simulink model "SVC_Simulation_new"  (R2024a)
settings: Solver=FixedStepDiscrete  StartTime=0.0  StopTime=0.6  FixedStep=Ts  RelTol=1e-3
model workspace (MAT data in the model file):
  Bcap = Simulink.Parameter
  Bcap.Value = 3.23
  Bcap.Complexity = 'real'
  Bcap.Dimensions = [1 1]
  Bcap.DataType = 'auto'
  Bind = Simulink.Parameter
  Bind.Value = -1.04
  Bind.Complexity = 'real'
  Bind.Dimensions = [1 1]
  Bind.DataType = 'auto'
  Bmax = Simulink.Parameter
  Bmax.Value = 3.23
  Bmax.Complexity = 'real'
  Bmax.Dimensions = [1 1]
  Bmax.DataType = 'auto'
  Bmin = Simulink.Parameter
  Bmin.Value = -1.04
  Bmin.Complexity = 'real'
  Bmin.Dimensions = [1 1]
  Bmin.DataType = 'auto'
  Bmmin_max = 0
  Bref = 0
  Ki = Simulink.Parameter
  Ki.Value = 800
  Ki.Complexity = 'real'
  Ki.Dimensions = [1 1]
  Ki.DataType = 'auto'
  Kp = Simulink.Parameter
  Kp.Value = 0
  Kp.Complexity = 'real'
  Kp.Dimensions = [1 1]
  Kp.DataType = 'auto'
  KpKi = 0
  OpMode = 1
  Ts = 5e-05
  Vref = 0
  Xs = 0
undefined symbols (not defined in the file or in its folder): D1, Delta, DiscIntNeverNeededParam
libraries: spsThreePhaseVIMeasurementLib x2, spsThreePhaseSeriesRLCLoadLib x1, spsThreePhaseTransformerTwoWindingsLib x1, spsThreePhaseSeriesRLCBranchLib x1, spsGroundLib x1, spsPLL3phLib x1, spsPositiveSequencePLLDrivenLib x1, spsThreePhaseProgrammableVoltageSourceLib x1, spsStairGeneratorLib x1, sps_lib x1
settings Model: ParameterArgumentNames=Bmmin_max,Bref,KpKi,OpMode,Ts,Vref,Xs  Creator=E370_  LastModifiedBy=E370_

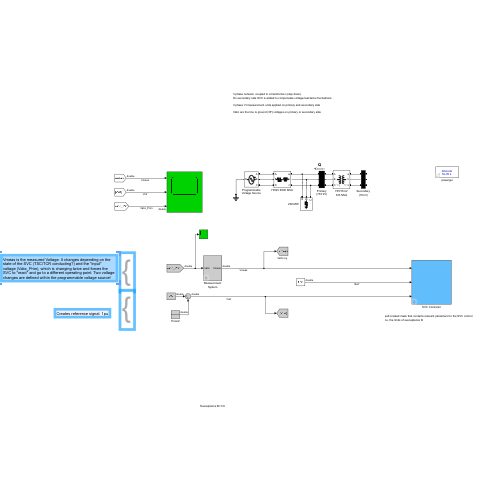
[thumbnail: Simulink's stored preview of the top-level diagram]
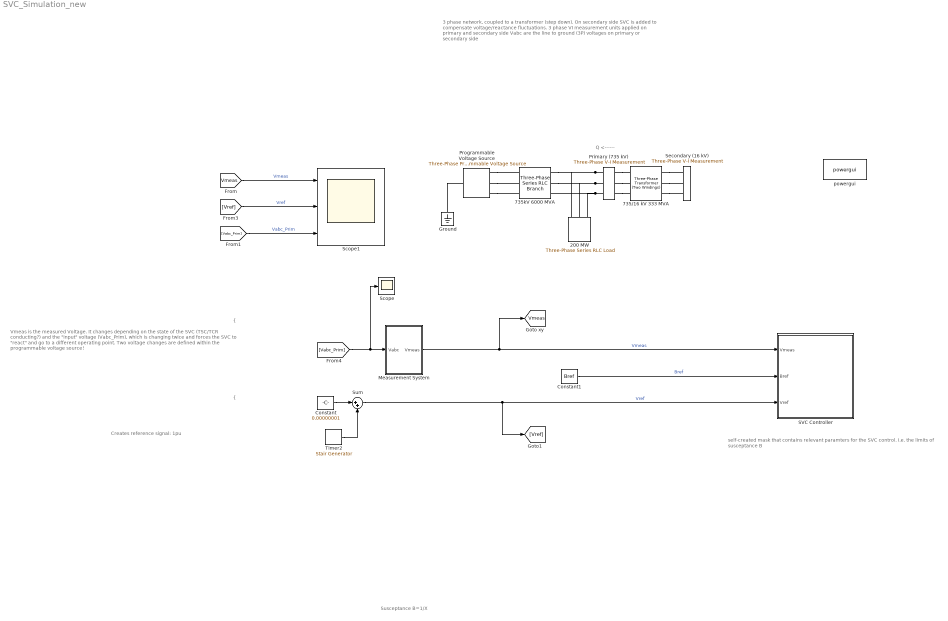
== system SVC_Simulation_new ==
  note: {
  note: Vmeas is the measured Voltage. It changes depending on the state of the SVC (TSC/TCR conducting?) and the "input" voltage (Vabc_Prim), which is changing twice and forces the SVC to "react" and go to a different operating point. Two voltage changes are defined within the programmable voltage source!
  note: self-created mask that contains relevant paramters for the SVC control.
      | I.e. the limits of susceptance B
  note: Susceptance B=1/X
  note: Creates reference signal: 1pu
  note: 3 phase network, coupled to a transformer (step down).
      | On secondary side SVC is added to compensate voltage/reactance fluctuations.
      |
      | 3 phase VI measurement units applied on primary and secondary side
      |
      | Vabc are the line to ground (3P) voltages on primary or secondary side
  note: Q
      | <------
  note: {
  200 MW : spsThreePhaseSeriesRLCLoadLib/Three-Phase Series RLC Load  LConnTagsString=A|B|C  Configuration=Y (grounded)  NominalVoltage=735e3  Vabc=[1e3 1e3 1e3]  Vabcp=[1e3 1e3 1e3]  NominalFrequency=60  UnbalancedPower=off  ActivePower=200e6  InductivePower=0  CapacitivePower=0  Pabc=[10e3 9e3 11e3]  QLabc=[100 90 110]  QCabc=[100 90 110]  Pabcp=[10e3 9e3 11e3]  QLabcp=[100 90 110]  QCabcp=[100 90 110]  Measurements=None  LoadType=constant Z
  735/16 kV 333 MVA : spsThreePhaseTransformerTwoWindingsLib/Three-Phase Transformer (Two Windings)  Winding1Connection=Yg  Winding2Connection=Delta (D1)  CoreType=Three single-phase transformers  SetSaturation=off  Hysteresis=off  DataFile='hysteresis'  SetInitialFlux=off  Measurements=None  UNITS=pu  NominalPower=[333e6 , 60 ]  Winding1=[735e3 , 0.15/30/2 , 0.15*0.7]  Winding2=[ 16e3 , 0.15/30/2, 0.15*0.3]  Rm=500  Lm=500  L0=0.5  Saturation="[ 0,0  ;  0.005,1.2  ;  1.0,1.4 ]"  InitialFluxes=[ 0.8 , -0.8 , 0.7 ]  BreakLoop=off  DiscreteSolver=Trapezoidal iterative  DataType=off  TransfoNumber=0
  "735kV 6000 MVA " : spsThreePhaseSeriesRLCBranchLib/Three-Phase Series RLC Branch  LConnTagsString=A|B|C  RConnTagsString=A|B|C  BranchType=RL  Resistance=735e3^2/6000e6/10  Inductance=735e3^2/6000e6/(2*pi*60)  Capacitance=1.0  Measurements=None
  Constant : Constant  Value=0.00000001
  Constant1 : Constant  Value=Bref
  Ground : spsGroundLib/Ground  LConnTagsString=a
  Measurement System : Subsystem  mask(SVC measurement system){Vnom=735e3, ParI=[735e3*0.9998 0 60], Ts=Ts}
      mask prompts: Vnom "Nominal voltage (volts rms ph-ph)"; ParI "Initial input: [ Mag (volts rms ph-ph)  Phase (degree) Freq (Hz) ]"; Ts "Sample time:"
      mask init:
      | Mag_Init=ParI(1)/Vnom;
      | Phase_Init=ParI(2);
      | Freq_Init=ParI(3);
  Primary (735 kV) : spsThreePhaseVIMeasurementLib/Three-Phase V-I Measurement  VoltageMeasurement=phase-to-ground  SetLabelV=on  LabelV=Vabc_Prim  Vpu=on  VpuLL=off  CurrentMeasurement=yes  SetLabelI=on  LabelI=Iabc_Prim  Ipu=on  Pbase=100e6  Vbase=735e3  OutputType=Magnitude  PhasorSimulation=off  PSBequivalent=0
  Programmable Voltage Source : spsThreePhaseProgrammableVoltageSourceLib/Three-Phase Programmable Voltage Source  PositiveSequence="[1.004*735e3 0  60]"  VariationEntity=Amplitude  VariationType=Table of time-amplitude pairs  VariationTypeAlt=Step  VariationStep=-0.3  VariationRate=0.5  VariationMagnitude=0.4  VariationFrequency=2  VariationTiming=[0.1 1.2]  VariationPhaseA=off  Amplitudes=[1.0 1.025 0.93 1.0 ]  TimeValues=[0 0.1 0.4 0.7]  HarmonicGeneration=off  HarmonicA=[3 0.2 -25 0]  HarmonicB="[2 0.15  35 2]"  Timing="[0.1  0.6]"  BusType=swing  Pref=0  Qref=0  Qmin=-inf  Qmax=inf
  SVC Controller : Subsystem  mask{Vref=1.0, KpKi=[ 0 800 ], Xs=0.01, Bmin_max=[ -1.04 3.23], Bref=0, Ts=Ts}
      mask prompts: Vref "reference voltage (pu):"; KpKi "regulator gains [Kp Ki]:"; Xs "droop"; Bmin_max "Min. and max. primary susceptances [ Bind Bcap] (pu/100MVA):"; Bref "susceptance Bref (pu/100MVA) (Var control mode):"; Ts "sample time (s):"
      mask DialogControl Control2 Prompt: Voltage Regulation Mode
      mask Display: color('red');
  Scope : Scope
  Scope1 : Scope  NumInputPorts=3
  Secondary (16 kV) : spsThreePhaseVIMeasurementLib/Three-Phase V-I Measurement  VoltageMeasurement=phase-to-phase  SetLabelV=on  LabelV=Vabc_Sec  Vpu=on  VpuLL=off  CurrentMeasurement=no  SetLabelI=off  LabelI=Iabc_Sec  Ipu=off  Pbase=100e6  Vbase=16e3  OutputType=Magnitude  PhasorSimulation=off  PSBequivalent=0
  Sum : Sum  Inputs=|++  SaturateOnIntegerOverflow=on
  Timer2 : spsStairGeneratorLib/Stair Generator  t="[ 0  0.4  0.6 ]"  e=[1 1 1 ]  Ts=Ts
  powergui : sps_lib/powergui  Priority=1  SimulationMode=Discrete  SampleTime=Ts  frequency=60  Iterations=50  frequencyindice=60  Pbase=100e6  ErrMax=1e-4  UnitsV=kV  UnitsW=MW  buscounter=0  FunctionMessages=off  echomessages=off  EnableUseOfTLC=off  CurrentSourceSwitches=off  DisableSnubberDevices=off  DisableRonSwitches=off  DisableVfSwitches=off  DisplayEquations=off  AutomaticDiscreteSolvers=off  SolverType=Tustin/Backward Euler (TBE)  Interpol=off  ExternalGateDelay=off  methode=off  Ts=100  x0status=blocks  SPID=on  SwTol=0  HookPort=off  NonlinearTolerance=1e-4  nMaxIteration=100  ContinueOnMaxIteration=off  RestoreLinks=warning  ResistiveCurrentMeasurement=off  Frange=[0:2:500]  Ylog=off  Xlog=on  ShowGrid=off  save=off  variable=ZData  structure=0  ZoomFFT=off  StartTime=0.0  cycles=1  DisplayStyle=1  fundamental=60  FreqAxis=off  MaxFrequency=1000  frequencyindicesteady=1  RmsSteady=1  display=off
  tag scope: Vmeas=global
  wires:
  [Vabc_Prim] -> Scope/1, Measurement System/1(Vabc)
  Timer2/1 -> Sum/2
  Constant/1 -> Sum/1
  [Vref] -> Scope1/2  "Vref"
  Constant1/1 -> SVC Controller/2(Bref)  "Bref"
  Measurement System/1(Vmeas) -> [Vmeas], SVC Controller/1(Vmeas)  "Vmeas"
  [Vmeas] -> Scope1/1  "Vmeas"
  Sum/1 -> SVC Controller/3(Vref), [Vref]  "Vref"
  [Vabc_Prim] -> Scope1/3  "Vabc_Prim"
  connections:
  Primary (735 kV)/LConn2 -- 200 MW/LConn2 -- "735kV 6000 MVA "/RConn2
  Primary (735 kV)/LConn3 -- 200 MW/LConn3 -- "735kV 6000 MVA "/RConn3
  Primary (735 kV)/LConn1 -- 200 MW/LConn1 -- "735kV 6000 MVA "/RConn1
  Primary (735 kV)/RConn3 -- 735/16 kV 333 MVA/LConn3
  Programmable Voltage Source/RConn1 -- "735kV 6000 MVA "/LConn1
  Primary (735 kV)/RConn1 -- 735/16 kV 333 MVA/LConn1
  Primary (735 kV)/RConn2 -- 735/16 kV 333 MVA/LConn2
  Programmable Voltage Source/RConn2 -- "735kV 6000 MVA "/LConn2
  Programmable Voltage Source/RConn3 -- "735kV 6000 MVA "/LConn3
  735/16 kV 333 MVA/RConn3 -- Secondary (16 kV)/LConn3
  Ground/LConn1 -- Programmable Voltage Source/LConn1
  735/16 kV 333 MVA/RConn2 -- Secondary (16 kV)/LConn2
  735/16 kV 333 MVA/RConn1 -- Secondary (16 kV)/LConn1

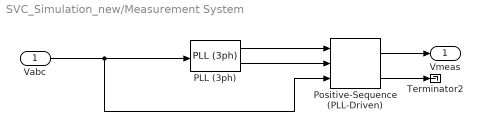
== system SVC_Simulation_new/Measurement System ==
  Vabc : Inport  PortDimensions=3
  PLL (3ph) : spsPLL3phLib/PLL (3ph)  Fmin=45  Par_Init=[Phase_Init Freq_Init]  ParK=[60 1400 0]  TcD=1e-4  MaxRateChangeFreq=12  FilterCutOffFreq=25  Ts=Ts  AGC=off
  Positive-Sequence (PLL-Driven) : spsPositiveSequencePLLDrivenLib/Positive-Sequence (PLL-Driven)  Finit=Freq_Init  Fmin=45  InInit=[Mag_Init 0]  Ts=Ts
  Terminator2 : Terminator
  Vmeas : Outport  VectorParamsAs1DForOutWhenUnconnected=off
  wires:
  PLL (3ph)/1 -> Positive-Sequence (PLL-Driven)/1
  PLL (3ph)/2 -> Positive-Sequence (PLL-Driven)/2
  Vabc/1 -> Positive-Sequence (PLL-Driven)/3, PLL (3ph)/1
  Positive-Sequence (PLL-Driven)/2 -> Terminator2/1
  Positive-Sequence (PLL-Driven)/1 -> Vmeas/1

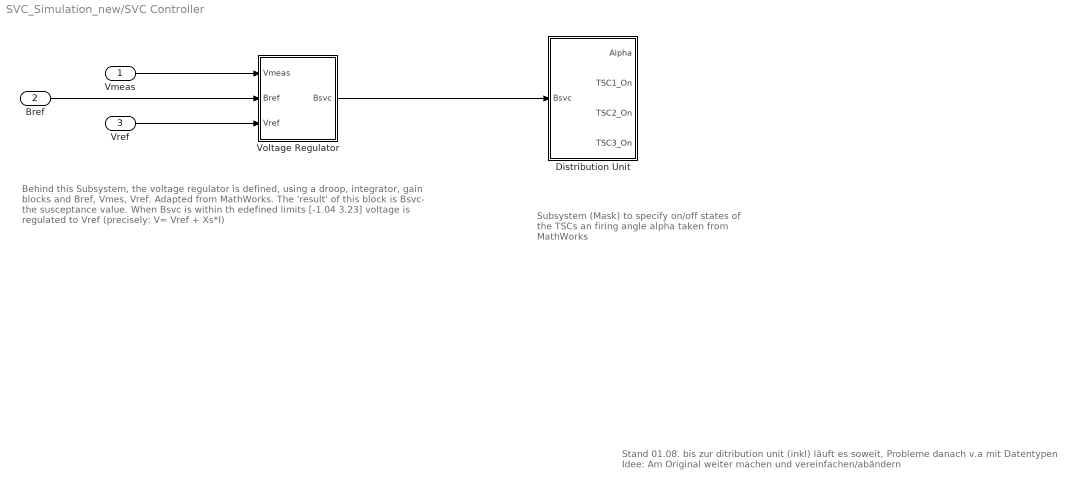
== system SVC_Simulation_new/SVC Controller ==
  note: Stand 01.08. bis zur ditribution unit (inkl) läuft es soweit, Probleme danach v.a mit Datentypen
      |
      | Idee: Am Original weiter machen und vereinfachen/abändern
  note: Subsystem (Mask) to specify on/off states
      | of the TSCs an firing angle alpha
      | taken from MathWorks
  note: Behind this Subsystem, the voltage regulator is defined, using a droop, integrator,
      | gain blocks and Bref, Vmes, Vref.
      | Adapted from MathWorks.
      | The 'result' of this block is Bsvc- the susceptance value.
      | When Bsvc is within th edefined limits [-1.04 3.23] voltage is regulated to Vref
      | (precisely: V= Vref + Xs*I)
  Vmeas : Inport
  Bref : Inport  Port=2  PortDimensions=1
  Vref : Inport  Port=3
  Distribution Unit : Subsystem  mask(Distribution Unit){ParNom=[333e6 60], Xf_xfo=0.15, Vsec_svc=16e3, L_TCR=18.7e-3, C_TSC=308.4e-6, L_TSC=1.13e-3, hyst_svc=0.1, Ts=Ts}
      mask prompts: ParNom "Transformer nominal power and frequency: [  P (VA)    Freq (Hz)  ]"; Xf_xfo "Transformer total leakage (pu/Pnom):"; Vsec_svc "Nominal secondary voltage (Volts rms ph-ph):"; L_TCR "TCR branch inductance (H):"; C_TSC "TSC branch capacitance (F):"; L_TSC "TSC branch inductance (H)"; hyst_svc "Hysteresis - Distribution unit (pu/100MVA):"; Ts "Sample time:"
      mask init:
      | Pnom_xfo=ParNom(1);
      | Freq=ParNom(2);
      | Bsec_pu100=100e6/Vsec_svc/Vsec_svc/3;
      | w=2*pi*Freq;
      | Bpu_TCR=-1/L_TCR/w/Bsec_pu100;
      | Bpu_TSC=1/(1/w/C_TSC-L_TSC*w)/Bsec_pu100;
      | B=1:-0.0025:0.0;
      | B=B';
      | for i=1:401,
      |       if B(i) <= 0,
      | 	ang = 0;
      |       elseif B(i) >= 1,
      | 	ang = pi;
      |       else,
      | 	a = pi; e = .0001;
      | 	da = a;
      | 	while abs(da)>e,
      | 		da = (pi*B(i)-a+sin(a))/(1-cos(a));
      | 		a = a + da;
      | 	end;
      | 	ang = a;
      |       end;
      |       A(i)=(180-ang*180/pi)/2+90;
      | end
      | A=A';
      | B=-B;
  Voltage Regulator : Subsystem
  wires:
  Bref/1 -> Voltage Regulator/2(Bref)
  Vmeas/1 -> Voltage Regulator/1(Vmeas)
  Vref/1 -> Voltage Regulator/3(Vref)
  Voltage Regulator/1(Bsvc) -> Distribution Unit/1(Bsvc)

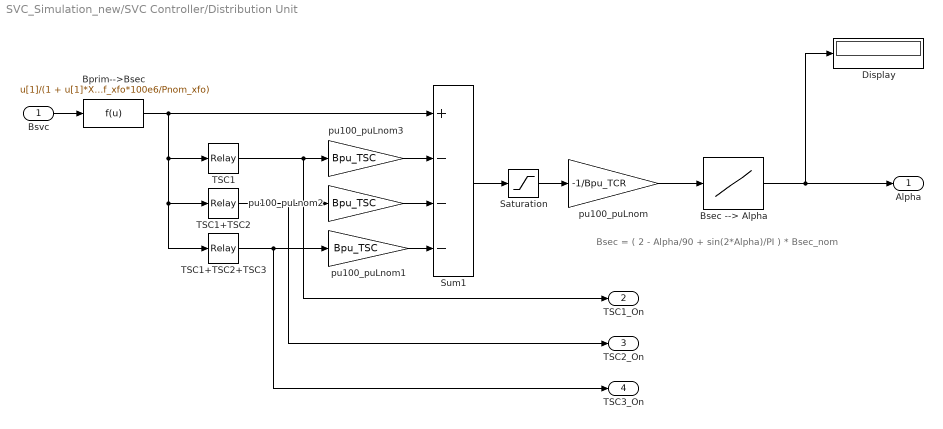
== system SVC_Simulation_new/SVC Controller/Distribution Unit ==
  note: Bsec = ( 2 - Alpha/90 + sin(2*Alpha)/PI ) * Bsec_nom
  Bsvc : Inport  PortDimensions=1
  Bprim-->Bsec : Fcn  Expr=u[1]/(1 + u[1]*Xf_xfo*100e6/Pnom_xfo)
  Bsec --> Alpha : Lookup_n-D  NumberOfTableDimensions=1  BreakpointsForDimension1=B  BreakpointsForDimension2=[0 571.55 685.8 800.15 914.4 1028.8 1143.1 1257.4 1371.7 1486 1600.3 1714.6 1828.9 1943.2 2057.5 2171.8 2286.1 2400.5 2514.7 2629.1 2743.3 2857.7 2971.9 3086.3 3200.5 3314.9 3429.2]  Table=A  InternalRulePriority=Speed  RndMeth=Simplest
  Display : Display
  Saturation : Saturate  UpperLimit=0  LowerLimit=Bpu_TCR
  Sum1 : Sum  Inputs=+---  InputSameDT=on  SaturateOnIntegerOverflow=on  OutDataTypeStr=Inherit: Same as first input
  TSC1 : Relay  OnSwitchValue=0  OffSwitchValue=-1 * hyst_svc
  TSC1+TSC2 : Relay  OnSwitchValue=0+ Bpu_TSC  OffSwitchValue=-1 * hyst_svc + Bpu_TSC
  TSC1+TSC2+TSC3 : Relay  OnSwitchValue=0+ 2*Bpu_TSC  OffSwitchValue=-1 * hyst_svc + 2*Bpu_TSC
  pu100_puLnom : Gain  Gain=-1/Bpu_TCR  SaturateOnIntegerOverflow=on  OutDataTypeStr=Inherit: Same as input  ParamDataTypeStr=Inherit: Same as input
  pu100_puLnom1 : Gain  Gain=Bpu_TSC  SaturateOnIntegerOverflow=on  OutDataTypeStr=Inherit: Same as input  ParamDataTypeStr=Inherit: Same as input
  pu100_puLnom2 : Gain  Gain=Bpu_TSC  SaturateOnIntegerOverflow=on  OutDataTypeStr=Inherit: Same as input  ParamDataTypeStr=Inherit: Same as input
  pu100_puLnom3 : Gain  Gain=Bpu_TSC  SaturateOnIntegerOverflow=on  OutDataTypeStr=Inherit: Same as input  ParamDataTypeStr=Inherit: Same as input
  Alpha : Outport  InitialOutput=0  VectorParamsAs1DForOutWhenUnconnected=off
  TSC1_On : Outport  Port=2  InitialOutput=0  VectorParamsAs1DForOutWhenUnconnected=off
  TSC2_On : Outport  Port=3  InitialOutput=0  VectorParamsAs1DForOutWhenUnconnected=off
  TSC3_On : Outport  Port=4  InitialOutput=0  VectorParamsAs1DForOutWhenUnconnected=off
  wires:
  TSC1/1 -> TSC1_On/1, pu100_puLnom3/1
  Sum1/1 -> Saturation/1
  TSC1+TSC2/1 -> TSC2_On/1, pu100_puLnom2/1
  TSC1+TSC2+TSC3/1 -> TSC3_On/1, pu100_puLnom1/1
  pu100_puLnom1/1 -> Sum1/4
  pu100_puLnom/1 -> Bsec --> Alpha/1
  Bsvc/1 -> Bprim-->Bsec/1
  Saturation/1 -> pu100_puLnom/1
  Bprim-->Bsec/1 -> TSC1+TSC2+TSC3/1, TSC1+TSC2/1, TSC1/1, Sum1/1
  Bsec --> Alpha/1 -> Display/1, Alpha/1
  pu100_puLnom2/1 -> Sum1/3
  pu100_puLnom3/1 -> Sum1/2

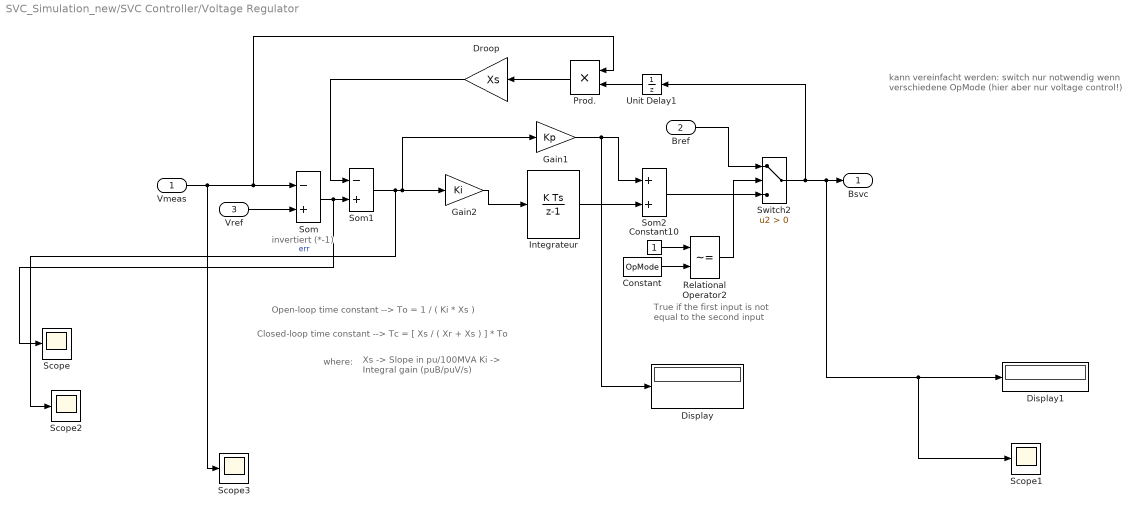
== system SVC_Simulation_new/SVC Controller/Voltage Regulator ==
  note: kann vereinfacht werden: switch nur notwendig
      | wenn verschiedene OpMode (hier aber nur voltage control!)
  note: True if the first input is not
      | equal to the second input
  note: where:
  note: Xs -> Slope in pu/100MVA
      |  Ki -> Integral gain (puB/puV/s)
  note: Open-loop time constant --> To = 1 / ( Ki * Xs )
  note: Closed-loop time constant --> Tc = [ Xs / ( Xr + Xs ) ] * To
  note: invertiert (*-1)
  Vmeas : Inport  PortDimensions=1
  Bref : Inport  Port=2  PortDimensions=1
  Vref : Inport  Port=3
  Constant : Constant  Value=OpMode
  Constant10 : Constant
  Display : Display
  Display1 : Display
  Droop : Gain  Gain=Xs  SaturateOnIntegerOverflow=on  OutDataTypeStr=Inherit: Same as input  ParamDataTypeStr=Inherit: Same as input
  Gain1 : Gain  Gain=Kp  SaturateOnIntegerOverflow=on  OutDataTypeStr=Inherit: Same as input  ParamDataTypeStr=Inherit: Same as input
  Gain2 : Gain  Gain=Ki  SaturateOnIntegerOverflow=on  OutDataTypeStr=Inherit: Same as input  ParamDataTypeStr=Inherit: Same as input
  Integrateur : DiscreteIntegrator  SampleTime=Ts  LimitOutput=on  UpperSaturationLimit=Bcap  LowerSaturationLimit=Bind  ICPrevOutput=DiscIntNeverNeededParam  ICPrevScaledInput=DiscIntNeverNeededParam
  Prod. : Product  InputSameDT=on  SaturateOnIntegerOverflow=on  OutDataTypeStr=Inherit: Same as first input
  Relational Operator2 : RelationalOperator  Operator=~=
  Scope{,1..3} (4 alike) : Scope
  Som : Sum  Inputs=-+  InputSameDT=on  SaturateOnIntegerOverflow=on  OutDataTypeStr=Inherit: Same as first input
  Som1 : Sum  Inputs=-+  InputSameDT=on  SaturateOnIntegerOverflow=on  OutDataTypeStr=Inherit: Same as first input
  Som2 : Sum  InputSameDT=on  SaturateOnIntegerOverflow=on  OutDataTypeStr=Inherit: Same as first input
  Switch2 : Switch  Criteria=u2 > Threshold
  Unit Delay1 : UnitDelay  SampleTime=Ts  HasFrameUpgradeWarning=on
  Bsvc : Outport  InitialOutput=0  VectorParamsAs1DForOutWhenUnconnected=off
  wires:
  Som1/1 -> Scope2/1, Gain2/1, Gain1/1  "err"
  Constant10/1 -> Relational Operator2/1
  Som/1 -> Scope/1, Som1/2
  Integrateur/1 -> Som2/2
  Prod./1 -> Droop/1
  Vref/1 -> Som/2
  Vmeas/1 -> Scope3/1, Prod./1, Som/1
  Droop/1 -> Som1/1
  Bref/1 -> Switch2/1
  Gain2/1 -> Integrateur/1
  Som2/1 -> Switch2/3
  Switch2/1 -> Scope1/1, Display1/1, Bsvc/1, Unit Delay1/1
  Constant/1 -> Relational Operator2/2
  Relational Operator2/1 -> Switch2/2
  Unit Delay1/1 -> Prod./2
  Gain1/1 -> Display/1, Som2/1
